simulink model "Simulator_DecMPC_v1"  (R2023a)
settings: Solver=ode45  StartTime=0  StopTime=86400  RelTol=1e-3
values from neighbouring files (symbols this model uses):
  A = Household_DecMPC(T_set, T_amb, Ts, K, Q, [NAME_SIMULATION '/' ADRESS_NMPC_A ], true)    [mainDecMPC_v1.m]
  B = Household_DecMPC(T_set, T_amb, Ts, K, Q, [NAME_SIMULATION '/' ADRESS_NMPC_B ], true)    [mainDecMPC_v1.m]
  C = Household_DecMPC(T_set, T_amb, Ts, K, Q, [NAME_SIMULATION '/' ADRESS_NMPC_C ], true)    [mainDecMPC_v1.m]
  K_m_dot = 0    [mainDecMPC_v1.m]
  K_temp = 0    [mainDecMPC_v1.m]
  m_dot_FEED_MAX = 20    [mainDecMPC_v1.m]
  m_dot_NOMINAL_BYP = 0.1 * m_dot_NOMINAL_FEED    (= 1)    [mainDecMPC_v1.m]
  m_dot_NOMINAL_FEED = 10    [mainDecMPC_v1.m]
  T_amb = 273    [mainDecMPC_v1.m]
  T_FEED_MAX = 370    [mainDecMPC_v1.m]
  T_FEED_MIN = 320    [mainDecMPC_v1.m]
  T_NOMINAL_FEED = 350    [mainDecMPC_v1.m]
  T_SP_RETURN = 310    [mainDecMPC_v1.m]
libraries: mpclib x3
settings Model: Creator=alex  LastModifiedBy=alex

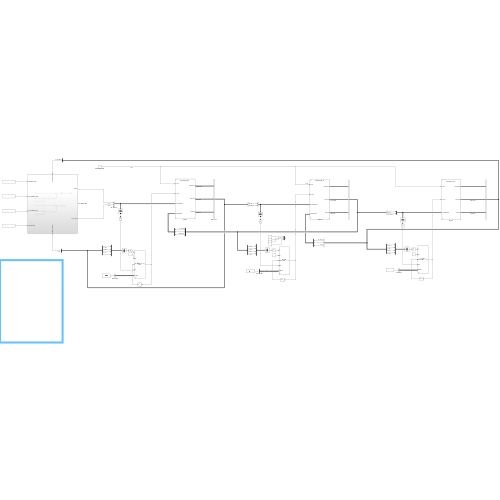
[thumbnail: Simulink's stored preview of the top-level diagram]
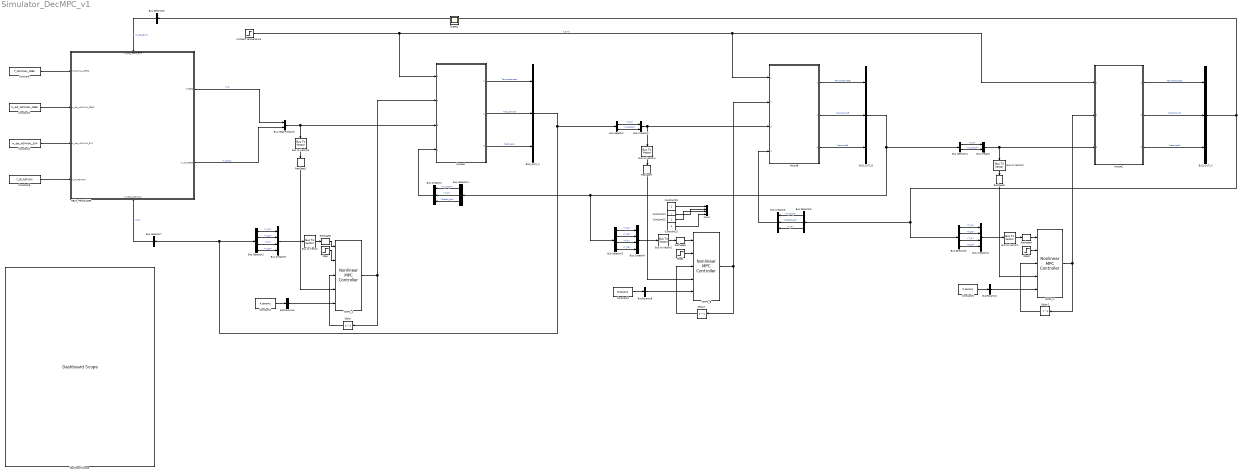
== system Simulator_DecMPC_v1 ==
  Ambient temperature : Step  Time=0  Before=T_amb  After=T_amb  SampleTime=0
  BUS_OUT_A : BusCreator  Inputs=3
  BUS_OUT_B : BusCreator  Inputs=3
  BUS_OUT_C : BusCreator  Inputs=3
  Bus Creator : BusCreator  Inputs=2
  Bus Creator10 : BusCreator  Inputs=4
  Bus Creator2 : BusCreator  Inputs=3
  Bus Creator3 : BusCreator  Inputs=2
  Bus Creator6 : BusCreator  Inputs=3
  Bus Creator8 : BusCreator  Inputs=4
  Bus Creator9 : BusCreator  Inputs=4
  Bus Heat Producer : BusCreator  Inputs=2
  Bus Selector : BusSelector  OutputSignals=TemperaturesA.T_O,mass_flowsA.m_dot_O
  Bus Selector1 : BusSelector  OutputSignals=mass_flowsB.m_dot_R,TemperaturesB.T_R,PressuresB.DeltaP_tot
  Bus Selector2 : BusSelector  OutputSignals=TemperaturesA.T_S1,TemperaturesA.T_S2,TemperaturesA.T_b,TemperaturesA.T_S3
  Bus Selector3 : BusSelector  OutputSignals=TemperaturesB.T_S1,TemperaturesB.T_S2,TemperaturesB.T_b,TemperaturesB.T_S3
  Bus Selector4 : BusSelector  OutputSignals=TemperaturesB.T_O,mass_flowsB.m_dot_O
  Bus Selector5 : BusSelector  OutputSignals=TemperaturesC.T_S1,TemperaturesC.T_S2,TemperaturesC.T_b,TemperaturesC.T_S3
  Bus Selector6 : BusSelector  OutputSignals=mass_flowsC.m_dot_R,PressuresC.DeltaP_tot,TemperaturesC.T_R
  Bus Selector7 : BusSelector  OutputSignals=TemperaturesA.T_R
  Bus Selector8 : BusSelector  OutputSignals=mass_flowsC.m_dot_BYP
  Bus to Vector{,1..5} (6 alike) : BusToVector
  BusParamsA : BusCreator  Inputs=1  OutDataTypeStr=Bus: BusParamsA  NonVirtualBus=on
      settings: InheritFromInputs=off
  BusParamsB : BusCreator  Inputs=1  OutDataTypeStr=Bus: BusParamsB  NonVirtualBus=on
      settings: InheritFromInputs=off
  BusParamsC : BusCreator  Inputs=1  OutDataTypeStr=Bus: BusParamsC  NonVirtualBus=on
      settings: InheritFromInputs=off
  Constant : Constant  Value=T_NOMINAL_FEED
  Constant1 : Constant  Value=A.params
  Constant2 : Constant  Value=m_dot_NOMINAL_FEED
  Constant{20..23} (4 alike) : Constant
  Constant3 : Constant  Value=B.params
  Constant4 : Constant  Value=m_dot_NOMINAL_BYP
  Constant5 : Constant  Value=C.params
  Constant6 : Constant  Value=T_SP_RETURN
  Dashboard Scope : DashboardScope
  Delay : Delay  DelayLength=1
  Delay1 : Delay  DelayLength=1
  Delay2 : Delay  DelayLength=1
  HEAT_PRODUCER : Subsystem
      settings: PortSchema="{\"entries\":[{\"content\":{\"sides\":[{\"content\":{\"connectorIds\":[\"In1\",\"In2\",\"In3\",\"In4\"]},\"type\":\"ConnectorPlacement.EquallySpacedRectSide\",\"uuid\":\"57470694-9f95-40c6-910d-c98b2fe962c6\"},{\"content\":{\"connectorIds\":[\"Out1\",\"Out2\"],\"side\":\"RIGHT\"},\"type\":\"ConnectorPlacement.EquallySpacedRectSide\",\"uuid\":\"ea169ea0-7e41-44df-a0d2-84b8273e8160\"},{\"content\":{\"connectorIds\":[\"In5\"],\"side\":\"TOP\"},\"type\":\"ConnectorPlacement.EquallySpacedRectSide\",\"uuid\":\"dd8e6ca4-5bfb-4619-87b5-e8cde4c1d523\"},{\"content\":{\"connectorIds\":[\"In6\"],\"side\":\"BOTTOM\"},\"type\":\"ConnectorPlacement.EquallySpacedRectSide\",\"uuid\":\"49c8c343-c48a-4638-bfea-a907688940c0\"}]},\"type\":\"ConnectorPlacement.EquallySpacedConnector\",\"uuid\":\"fcf76c0f-e8b9-4e64-954e-173ccd5a3c51\"}],\"packageUris\":[\"http://schema.mathworks.com/mf0/Connector/R2020b\"],\"version\":\"1.0\"}"
  HouseA : Subsystem  ReferencedSubsystem=Simulator_MID_v4  rho=971  c_p=4179  pi=3.14151  f_Darcy=0.025  L_F=40  D_F=0.4  h_F=1.5  D_S1=0.1  L_S1=5  h_S1=1.5  D_S2=0.05  L_S2=50  h_S2=30  D_S3=0.4  L_S3=5  h_S3=1.5  D_R=0.4  L_R=40  h_R=1.5  C_b=3000000  A_b=100  h_b=1.5  L_BYP=3  D_BYP=0.1  h_BYP=1.5  T_F_0=283  T_S1_0=283  T_S2_0=283  T_S3_0=283  T_b_0=286  T_R_0=283  T_BYP_0=283
  HouseB : Subsystem  ReferencedSubsystem=Simulator_MID_v4  rho=971  c_p=4179  pi=3.14151  f_Darcy=0.025  L_F=40  D_F=0.4  h_F=1.5  D_S1=0.1  L_S1=5  h_S1=1.5  D_S2=0.05  L_S2=50  h_S2=30  D_S3=0.4  L_S3=5  h_S3=1.5  D_R=0.4  L_R=40  h_R=1.5  C_b=3000000  A_b=100  h_b=1.5  L_BYP=3  D_BYP=0.1  h_BYP=1.5  T_F_0=283  T_S1_0=283  T_S2_0=283  T_S3_0=283  T_b_0=286  T_R_0=283  T_BYP_0=283
  HouseC : Subsystem  ReferencedSubsystem=Simulator_BYP_v4  rho=971  rho_air=971  c_p=4179  c_p_air=4179  pi=3.14151  f_Darcy=0.025  L_F=40  D_F=0.4  h_F=1.5  D_S1=0.1  L_S1=5  h_S1=1.5  D_S2=0.05  L_S2=50  h_S2=30  D_S3=0.4  L_S3=5  h_S3=0.4  D_R=0.4  L_R=40  h_R=1.5  C_b=3000000  A_b=100  h_b=1.5  D_BYP=0.1  L_BYP=3  h_BYP=1.5  T_F_0=283  T_S1_0=283  T_S2_0=283  T_S3_0=283  T_b_0=286  T_R_0=283  T_BYP_0=283
  Mux4 : Mux
  NMPC_A : mpclib/Nonlinear MPC Controller  nlmpcobj=A.nlobj  UseObjectTs=on  UseMEX=off  md_enabled=on  mvtarget_enabled=off  param_enabled=on  cost_enabled=off  mvseq_enabled=off  stateseq_enabled=off  ovseq_enabled=off  slack_enabled=off  status_enabled=off  ov_min=off  ov_max=off  mv_min=off  mv_max=off  mvrate_min=off  mvrate_max=off  state_min=off  state_max=off  ov_weight=off  mv_weight=off  mvrate_weight=off  ecr_weight=off  nlp_initialize=off
  NMPC_B : mpclib/Nonlinear MPC Controller  nlmpcobj=B.nlobj  UseObjectTs=on  UseMEX=off  md_enabled=on  mvtarget_enabled=off  param_enabled=on  cost_enabled=off  mvseq_enabled=off  stateseq_enabled=off  ovseq_enabled=off  slack_enabled=off  status_enabled=off  ov_min=off  ov_max=off  mv_min=off  mv_max=off  mvrate_min=off  mvrate_max=off  state_min=off  state_max=off  ov_weight=off  mv_weight=off  mvrate_weight=off  ecr_weight=off  nlp_initialize=off
  NMPC_C : mpclib/Nonlinear MPC Controller  nlmpcobj=C.nlobj  UseObjectTs=on  UseMEX=off  md_enabled=on  mvtarget_enabled=off  param_enabled=on  cost_enabled=off  mvseq_enabled=off  stateseq_enabled=off  ovseq_enabled=off  slack_enabled=off  status_enabled=off  ov_min=off  ov_max=off  mv_min=off  mv_max=off  mvrate_min=off  mvrate_max=off  state_min=off  state_max=off  ov_weight=off  mv_weight=off  mvrate_weight=off  ecr_weight=off  nlp_initialize=off
  Reshape1 : Reshape  OutputDimensionality=Customize  OutputDimensions=[1,2]
  Reshape3 : Reshape  OutputDimensionality=Customize  OutputDimensions=[1,2]
  Reshape4 : Reshape  OutputDimensionality=Customize  OutputDimensions=[4,1]
  Reshape5 : Reshape  OutputDimensionality=Customize  OutputDimensions=[4,1]
  Reshape6 : Reshape  OutputDimensionality=Customize  OutputDimensions=[4,1]
  Reshape7 : Reshape  OutputDimensionality=Customize  OutputDimensions=[1,2]
  Step : Step  Time=360  Before=360  After=0  SampleTime=0
  Step1 : Step  Time=360  Before=360  After=0  SampleTime=0
  Step2 : Step  Time=360  Before=360  After=0  SampleTime=0
  Scope1 : Scope
  wires:
  HouseA/1 -> BUS_OUT_A/1  "TemperaturesA"
  HouseA/2 -> BUS_OUT_A/2  "mass_flowsA"
  HouseA/3 -> BUS_OUT_A/3  "PressuresA"
  Ambient temperature/1 -> HouseA/1, HouseC/1, HouseB/1  "T_amb"
  HouseB/1 -> BUS_OUT_B/1  "TemperaturesB"
  HouseB/2 -> BUS_OUT_B/2  "mass_flowsB"
  HouseB/3 -> BUS_OUT_B/3  "PressuresB"
  Bus Selector1/1 -> Bus Creator2/1  "<m_dot_R>"
  Bus Selector1/2 -> Bus Creator2/2  "<T_R>"
  Bus Selector1/3 -> Bus Creator2/3  "<DeltaP_tot>"
  Bus Creator2/1 -> HouseA/4
  Bus Creator3/1 -> HouseB/3, Bus to Vector4/1
  BUS_OUT_A/1 -> Bus Selector/1, Bus Selector7/1, Bus Selector2/1
  Bus Selector/2 -> Bus Creator3/2  "<m_dot_O>"
  Bus Heat Producer/1 -> HouseA/3, Bus to Vector5/1
  Bus Creator6/1 -> HouseB/4
  Bus Selector6/3 -> Bus Creator6/3  "<T_R>"
  Bus Selector6/2 -> Bus Creator6/2  "<DeltaP_tot>"
  Bus Selector6/1 -> Bus Creator6/1  "<m_dot_R>"
  HouseC/3 -> BUS_OUT_C/3  "PressuresC"
  HouseC/2 -> BUS_OUT_C/2  "mass_flowsC"
  HouseC/1 -> BUS_OUT_C/1  "TemperaturesC"
  NMPC_C/1 -> HouseC/2, Delay2/1
  NMPC_A/1 -> HouseA/2, Delay/1
  Bus Selector2/1 -> Bus Creator8/1  "<T_S1>"
  Bus Selector2/2 -> Bus Creator8/2  "<T_S2>"
  Bus Selector2/3 -> Bus Creator8/3  "<T_b>"
  Bus Selector2/4 -> Bus Creator8/4  "<T_S3>"
  Bus Creator8/1 -> Bus to Vector/1
  Delay/1 -> NMPC_A/3
  BusParamsA/1 -> NMPC_A/5
  Constant1/1 -> BusParamsA/1
  Bus Selector3/2 -> Bus Creator9/2  "<T_S2>"
  Bus Selector3/4 -> Bus Creator9/4  "<T_S3>"
  Bus Selector3/1 -> Bus Creator9/1  "<T_S1>"
  NMPC_B/1 -> Delay1/1, HouseB/2
  BusParamsB/1 -> NMPC_B/5
  Bus Selector3/3 -> Bus Creator9/3  "<T_b>"
  Bus Creator9/1 -> Bus to Vector1/1
  Delay1/1 -> NMPC_B/3
  Bus Selector/1 -> Bus Creator3/1  "<T_O>"
  Constant3/1 -> BusParamsB/1
  Bus Selector5/2 -> Bus Creator10/2  "<T_S2>"
  BusParamsC/1 -> NMPC_C/5
  Bus Selector5/4 -> Bus Creator10/4  "<T_S3>"
  Bus Selector5/3 -> Bus Creator10/3  "<T_b>"
  Bus Creator10/1 -> Bus to Vector2/1
  Delay2/1 -> NMPC_C/3
  Bus Selector5/1 -> Bus Creator10/1  "<T_S1>"
  Constant5/1 -> BusParamsC/1
  Constant/1 -> HEAT_PRODUCER/1(T_NOMINAL_FEED)
  Constant2/1 -> HEAT_PRODUCER/2(m_dot_NOMINAL_FEED)
  Constant4/1 -> HEAT_PRODUCER/3(m_dot_NOMINAL_BYP)
  Constant6/1 -> HEAT_PRODUCER/4(T_SP_RETURN)
  Bus Selector7/1 -> HEAT_PRODUCER/6(T_MEAS_RETURN)  "<T_R>"
  HEAT_PRODUCER/2(m_dot_FEED) -> Bus Heat Producer/2  "m_dot_O"
  HEAT_PRODUCER/1(T_FEED) -> Bus Heat Producer/1  "T_O"
  Bus Creator/1 -> HouseC/3, Bus to Vector3/1
  BUS_OUT_B/1 -> Bus Selector4/1, Bus Selector3/1, Bus Selector1/1
  Step/1 -> NMPC_A/2
  Bus Selector4/2 -> Bus Creator/2  "<m_dot_O>"
  Bus Selector4/1 -> Bus Creator/1  "<T_O>"
  Bus to Vector3/1 -> Reshape3/1
  Constant20/1 -> Mux4/1
  Constant21/1 -> Mux4/2
  Constant22/1 -> Mux4/3
  Constant23/1 -> Mux4/4
  Reshape3/1 -> NMPC_C/4
  Bus to Vector2/1 -> Reshape4/1
  Reshape4/1 -> NMPC_C/1
  Bus to Vector1/1 -> Reshape5/1
  Reshape5/1 -> NMPC_B/1
  Bus to Vector/1 -> Reshape6/1
  Reshape6/1 -> NMPC_A/1
  Bus to Vector4/1 -> Reshape7/1
  Reshape7/1 -> NMPC_B/4
  Bus Selector8/1 -> HEAT_PRODUCER/5(m_dot_MEAS_BYP)  "<m_dot_BYP>"
  BUS_OUT_C/1 -> Bus Selector6/1, Bus Selector5/1, Bus Selector8/1
  Reshape1/1 -> NMPC_A/4
  Bus to Vector5/1 -> Reshape1/1
  Step1/1 -> NMPC_B/2
  Step2/1 -> NMPC_C/2

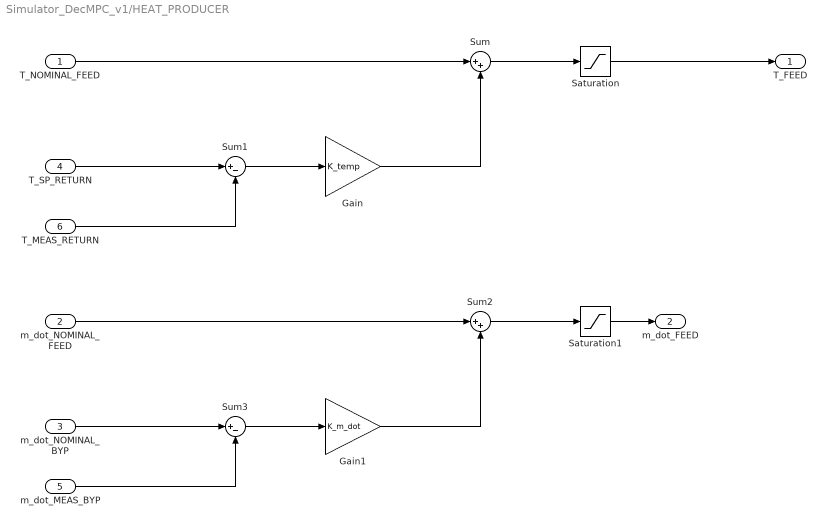
== system Simulator_DecMPC_v1/HEAT_PRODUCER ==
  T_NOMINAL_FEED : Inport
  m_dot_NOMINAL_FEED : Inport  Port=2
  m_dot_NOMINAL_BYP : Inport  Port=3
  T_SP_RETURN : Inport  Port=4
  m_dot_MEAS_BYP : Inport  Port=5
  T_MEAS_RETURN : Inport  Port=6
  Gain : Gain  Gain=K_temp
  Gain1 : Gain  Gain=K_m_dot
  Saturation : Saturate  UpperLimit=T_FEED_MAX  LowerLimit=T_FEED_MIN
  Saturation1 : Saturate  UpperLimit=m_dot_FEED_MAX  LowerLimit=0
  Sum : Sum  Inputs=|++
  Sum1 : Sum  Inputs=|+-
  Sum2 : Sum  Inputs=|++
  Sum3 : Sum  Inputs=|+-
  T_FEED : Outport
  m_dot_FEED : Outport  Port=2
  wires:
  T_MEAS_RETURN/1 -> Sum1/2
  Gain/1 -> Sum/2
  T_NOMINAL_FEED/1 -> Sum/1
  m_dot_NOMINAL_BYP/1 -> Sum3/1
  Sum/1 -> Saturation/1
  T_SP_RETURN/1 -> Sum1/1
  Sum1/1 -> Gain/1
  m_dot_MEAS_BYP/1 -> Sum3/2
  Gain1/1 -> Sum2/2
  Sum3/1 -> Gain1/1
  m_dot_NOMINAL_FEED/1 -> Sum2/1
  Saturation/1 -> T_FEED/1
  Saturation1/1 -> m_dot_FEED/1
  Sum2/1 -> Saturation1/1
